simulink model "MicrogridControl"  (R2025b)
settings: Solver=VariableStepAuto  StartTime=0.0  StopTime=8  FixedStep=Ts  RelTol=1e-3
PreLoadFcn:
  | NormalOperation;
  | MicrogridControlParam;
undefined symbols (not defined in the file): base, bessModeInitial, bessSystem, bessVoltage, breakerStatus, DiscIntNeverNeededParam, ee_sli_rtmsupport, event, gcbh, generator, gflInverter, gfmInverter, Inertia, lineInductance, lineResistance, machine, plannedIsland, pmsm, powerLimit, powerQuality, PV, PVInverter, ref, resync, solar, solarInsolationChange, systemFrequency, Ts, windController, windSystem, windTurbine
libraries: nesl_utility x234, ee_lib x174, fl_lib x143, eeGeneralControl x137, simulink x78, eeTransforms x47, slpidlib x23, nesl_utility_internal x12, eePwmGenerator x9, eeSinusoidalMeasurementV2 x9, custom_lib x7, batteryecm_lib x6
(part 24 of 25)

== system MicrogridControl/Solar/Solar Plant Integrated1/Detailed/PV Plant & Controller/Controller/Power Reference/Power Reference Controller/Power Reference Controller/Current_controller ==
  id-ref : Inport
  ipvd : Inport  Port=2
  iqref : Inport  Port=3
  iq : Inport  Port=4
  Vd : Inport  Port=5
  Vq : Inport  Port=6
  Constant4 : Constant  Value=0
  Gain1 : Gain  Gain=2*1*pi*60*L/zbase
  Gain2 : Gain  Gain=2*1*pi*60*L/zbase
  Mux1 : Mux  Inputs=3
  PID Controller : slpidlib/PID Controller  Controller=PID  Form=Parallel  TimeDomain=Discrete-time  UseExternalTs=off  SampleTime=-1  IntegratorMethod=Forward Euler  FilterMethod=Forward Euler  ControllerParametersSource=internal  P=Kpic  I=Kiic  UseKiTs=off  D=Kd  UseExternalDerivativeSource=off  N=100  UseFilter=on  TunerSelectOption=Transfer Function Based (PID Tuner App)  InitialConditionSource=internal  InitialConditionForIntegrator=0  InitialConditionForFilter=0  DifferentiatorICPrevScaledInput=0  ExternalReset=none  TrackingMode=off  Kt=1  LimitOutput=on  SatLimitsSource=internal  UpperSaturationLimit=3  LowerSaturationLimit=-3  LinearizeAsGain=on  AntiWindupMode=clamping  Kb=1  LimitIntegrator=on  UpperIntegratorSaturationLimit=3  LowerIntegratorSaturationLimit=-3  POutMin=[]  POutMax=[]  IOutMin=[]  IOutMax=[]  DOutMin=[]  DOutMax=[]  NOutMin=[]  NOutMax=[]  SumOutMin=[]  SumOutMax=[]  SaturationOutMin=[]  SaturationOutMax=[]  PParamMin=[]  PParamMax=[]  IParamMin=[]  IParamMax=[]  DParamMin=[]  DParamMax=[]  NParamMin=[]  NParamMax=[]  KbParamMin=[]  KbParamMax=[]  KtParamMin=[]  KtParamMax=[]  KbOutMin=[]  KbOutMax=[]  KtOutMin=[]  KtOutMax=[]  IntegratorOutMin=[]  IntegratorOutMax=[]  FilterOutMin=[]  FilterOutMax=[]  SumI1OutMin=[]  SumI1OutMax=[]  SumI2OutMin=[]  SumI2OutMax=[]  SumI3OutMin=[]  SumI3OutMax=[]  SumI4OutMin=[]  SumI4OutMax=[]  SumDOutMin=[]  SumDOutMax=[]  DifferentiatorOutMin=[]  DifferentiatorOutMax=[]  FilterDiffOutCoefMin=[]  FilterDiffOutCoefMax=[]  ReciprocalOutMin=[]  ReciprocalOutMax=[]  SumDenOutMin=[]  SumDenOutMax=[]  SumNumOutMin=[]  SumNumOutMax=[]  DivideOutMin=[]  DivideOutMax=[]  UdiffTsProdOutMin=[]  UdiffTsProdOutMax=[]  NTsProdOutMin=[]  NTsProdOutMax=[]  UintegralTsProdOutMin=[]  UintegralTsProdOutMax=[]  UngainTsProdOutMin=[]  UngainTsProdOutMax=[]  ClampingZeroOutDataTypeStr=Inherit: Inherit via back propagation  ClampingZeroOutMin=[]  ClampingZeroOutMax=[]  FilterDenConstantOutDataTypeStr=Inherit: Inherit via back propagation  FilterDenConstantOutMin=[]  FilterDenConstantOutMax=[]  PCopyOutDataTypeStr=Inherit: Inherit via back propagation  PCopyOutMin=[]  PCopyOutMax=[]  NCopyOutDataTypeStr=Inherit: Inherit via back propagation  NCopyOutMin=[]  NCopyOutMax=[]  IntegratorContinuousStateAttributes=''  IntegratorStateMustResolveToSignalObject=off  IntegratorRTWStateStorageClass=Auto  FilterContinuousStateAttributes=''  FilterStateMustResolveToSignalObject=off  FilterRTWStateStorageClass=Auto  ParallelPVariant=InternalParameters  IdealPVariant=Disabled  IVariant=InternalParameters  DVariant=InternalParameters  IntegratorVariant=Discrete  SatVariant=Enabled  AWVariant=DiscClampingParallel  PCopyVariant=Disabled  TRVariant=Disabled  FdbkBlocksVariant=Forward  IdealPFdbkVariant=Disabled  SatFdbkVariant=Disabled  DerivativeFilterVariant=ForwardEulerFilter  NVariant=InternalParameters  NCopyVariant=Disabled  FilterICVariant=InternalICsFilter  IntegratorICVariant=InternalICs  ExternalResetVariant=Disabled  TRSumVariant=Passthrough  SumFdbkVariant=Disabled  SumVariant=Sum_PID  TsampFilterVariant=InternalTs  TsampNgainVariant=Passthrough  TsampIntegralVariant=Disabled_SignalSpec  ExternalSaturationOutDataTypeStr=Inherit: Same as second input  DerivativeSourceVariant=ErrorSignal  PreIntVariant=InternalPreInt
  PID Controller1 : slpidlib/PID Controller  Controller=PID  Form=Parallel  TimeDomain=Discrete-time  UseExternalTs=off  SampleTime=-1  IntegratorMethod=Forward Euler  FilterMethod=Forward Euler  ControllerParametersSource=internal  P=Kpic  I=Kiic  UseKiTs=off  D=Kd  UseExternalDerivativeSource=off  N=100  UseFilter=on  TunerSelectOption=Transfer Function Based (PID Tuner App)  InitialConditionSource=internal  InitialConditionForIntegrator=0  InitialConditionForFilter=0  DifferentiatorICPrevScaledInput=0  ExternalReset=none  TrackingMode=off  Kt=1  LimitOutput=on  SatLimitsSource=internal  UpperSaturationLimit=3  LowerSaturationLimit=-3  LinearizeAsGain=on  AntiWindupMode=clamping  Kb=1  LimitIntegrator=on  UpperIntegratorSaturationLimit=3  LowerIntegratorSaturationLimit=-3  POutMin=[]  POutMax=[]  IOutMin=[]  IOutMax=[]  DOutMin=[]  DOutMax=[]  NOutMin=[]  NOutMax=[]  SumOutMin=[]  SumOutMax=[]  SaturationOutMin=[]  SaturationOutMax=[]  PParamMin=[]  PParamMax=[]  IParamMin=[]  IParamMax=[]  DParamMin=[]  DParamMax=[]  NParamMin=[]  NParamMax=[]  KbParamMin=[]  KbParamMax=[]  KtParamMin=[]  KtParamMax=[]  KbOutMin=[]  KbOutMax=[]  KtOutMin=[]  KtOutMax=[]  IntegratorOutMin=[]  IntegratorOutMax=[]  FilterOutMin=[]  FilterOutMax=[]  SumI1OutMin=[]  SumI1OutMax=[]  SumI2OutMin=[]  SumI2OutMax=[]  SumI3OutMin=[]  SumI3OutMax=[]  SumI4OutMin=[]  SumI4OutMax=[]  SumDOutMin=[]  SumDOutMax=[]  DifferentiatorOutMin=[]  DifferentiatorOutMax=[]  FilterDiffOutCoefMin=[]  FilterDiffOutCoefMax=[]  ReciprocalOutMin=[]  ReciprocalOutMax=[]  SumDenOutMin=[]  SumDenOutMax=[]  SumNumOutMin=[]  SumNumOutMax=[]  DivideOutMin=[]  DivideOutMax=[]  UdiffTsProdOutMin=[]  UdiffTsProdOutMax=[]  NTsProdOutMin=[]  NTsProdOutMax=[]  UintegralTsProdOutMin=[]  UintegralTsProdOutMax=[]  UngainTsProdOutMin=[]  UngainTsProdOutMax=[]  ClampingZeroOutDataTypeStr=Inherit: Inherit via back propagation  ClampingZeroOutMin=[]  ClampingZeroOutMax=[]  FilterDenConstantOutDataTypeStr=Inherit: Inherit via back propagation  FilterDenConstantOutMin=[]  FilterDenConstantOutMax=[]  PCopyOutDataTypeStr=Inherit: Inherit via back propagation  PCopyOutMin=[]  PCopyOutMax=[]  NCopyOutDataTypeStr=Inherit: Inherit via back propagation  NCopyOutMin=[]  NCopyOutMax=[]  IntegratorContinuousStateAttributes=''  IntegratorStateMustResolveToSignalObject=off  IntegratorRTWStateStorageClass=Auto  FilterContinuousStateAttributes=''  FilterStateMustResolveToSignalObject=off  FilterRTWStateStorageClass=Auto  ParallelPVariant=InternalParameters  IdealPVariant=Disabled  IVariant=InternalParameters  DVariant=InternalParameters  IntegratorVariant=Discrete  SatVariant=Enabled  AWVariant=DiscClampingParallel  PCopyVariant=Disabled  TRVariant=Disabled  FdbkBlocksVariant=Forward  IdealPFdbkVariant=Disabled  SatFdbkVariant=Disabled  DerivativeFilterVariant=ForwardEulerFilter  NVariant=InternalParameters  NCopyVariant=Disabled  FilterICVariant=InternalICsFilter  IntegratorICVariant=InternalICs  ExternalResetVariant=Disabled  TRSumVariant=Passthrough  SumFdbkVariant=Disabled  SumVariant=Sum_PID  TsampFilterVariant=InternalTs  TsampNgainVariant=Passthrough  TsampIntegralVariant=Disabled_SignalSpec  ExternalSaturationOutDataTypeStr=Inherit: Same as second input  DerivativeSourceVariant=ErrorSignal  PreIntVariant=InternalPreInt
  Saturation : Saturate  UpperLimit=1.2  LowerLimit=-1.2
  Saturation1 : Saturate  UpperLimit=1.2  LowerLimit=-1.2
  Scope : Scope  NumInputPorts=2
      settings: ActiveDisplayYMinimum=0.49995  ActiveDisplayYMaximum=0.50039
  Scope1 : Scope  NumInputPorts=2
      settings: ActiveDisplayYMinimum=-1  ActiveDisplayYMaximum=1  DataLoggingVariableName=ScopeData2
  Scope2 : Scope  NumInputPorts=3
      settings: ActiveDisplayYMinimum=0.92426  ActiveDisplayYMaximum=1.0261  DataLoggingVariableName=ScopeData2
  Sum1 : Sum  Inputs=|+-
  Sum3 : Sum  Inputs=|++-
  Sum4 : Sum  Inputs=|+++
  Sum5 : Sum  Inputs=|+-
  mdq0 : Outport
  wires:
  Vd/1 -> Sum3/1, Scope2/1
  Saturation1/1 -> Mux1/2
  Saturation/1 -> Mux1/1
  iqref/1 -> Sum5/1, Scope1/1
  Mux1/1 -> mdq0/1
  Sum4/1 -> [Eq], Saturation1/1
  PID Controller1/1 -> Sum4/1
  Sum5/1 -> PID Controller1/1
  Constant4/1 -> Mux1/3
  Sum1/1 -> PID Controller/1
  iq/1 -> Sum5/2, Gain2/1, Scope1/2
  Vq/1 -> Sum4/2
  Gain1/1 -> Sum4/3
  id-ref/1 -> Sum1/1, Scope/1
  ipvd/1 -> Sum1/2, Gain1/1, Scope/2
  Gain2/1 -> Sum3/3, Scope2/3
  Sum3/1 -> [Ed], Saturation/1
  PID Controller/1 -> Sum3/2, Scope2/2

== system MicrogridControl/Solar/Solar Plant Integrated1/Detailed/PV Plant & Controller/Controller/Power Reference/Power Reference Controller/Power Reference Controller/Reference Current ==
  note: Avoid division by zero during start
  note: Current Limiters
  V-mag : Inport
  LVRT_iq : Inport  Port=2
  PRef : Inport  Port=3
  QRef : Inport  Port=4
  Constant1 : Constant
  Constant3 : Constant  Value=Imax
  Current limits : Subsystem
  Refernce id generation : Subsystem
  Refernce iq generation : Subsystem
  Switch : Switch  Criteria=u2 ~= 0  SaturateOnIntegerOverflow=off  InputSameDT=off
  Unit Delay1 : UnitDelay  SampleTime=Ts  HasFrameUpgradeWarning=on
  Unit Delay3 : UnitDelay  SampleTime=Ts  HasFrameUpgradeWarning=on
  id_ref : Outport
  iq_ref : Outport  Port=2
  wires:
  Current limits/2(iubd) -> Refernce id generation/2(ubid)
  PRef/1 -> Refernce id generation/3(PRef)
  QRef/1 -> Refernce iq generation/4(Q_ref)
  Constant1/1 -> Switch/3
  Switch/1 -> Refernce iq generation/2(V_mag), Refernce id generation/1(V_mag)
  V-mag/1 -> Switch/2, Switch/1
  LVRT_iq/1 -> Refernce iq generation/3(LVRT_iq)
  Refernce iq generation/1(iq_ref) -> iq_ref/1, Unit Delay1/1
  Refernce id generation/1(id_ref) -> Unit Delay3/1, id_ref/1
  Constant3/1 -> Current limits/1(Imax)
  Unit Delay3/1 -> Current limits/3(idref)
  Current limits/1(iubq) -> Refernce iq generation/1(ubiq)
  Unit Delay1/1 -> Current limits/2(iqref)

== system MicrogridControl/Wind Farm/Wind Plant Integrated/Detailed/Wind Turbine and Converters/Wind Controller/Wind Grid-side Converter Controller/DC voltage controller & current reference/Subsystem1/V_dc_Controller1 ==
  Wind_plant1 : Inport
  In2 : Inport  Port=2
  Gain : Gain  Gain=1/Vdc
  PI : Subsystem
  Sum : Sum  Inputs=|+-
  Out1 : Outport
  wires:
  PI/1(Out2) -> Out1/1
  Gain/1 -> PI/1(Input)
  Sum/1 -> Gain/1
  In2/1 -> Sum/2
  Wind_plant1/1 -> Sum/1

== system MicrogridControl/Wind Farm/Wind Plant Integrated/Detailed/Wind Turbine and Converters/Wind Plant/Back-to-Back Converters/Switching/Grid Side Converter/Pulse Generation1 ==
  G : Inport
  Constant : Constant  Value=5
  Subtract : Sum  Inputs=-+
  G1 : Outport  VectorParamsAs1DForOutWhenUnconnected=off
  G2 : Outport  Port=2  VectorParamsAs1DForOutWhenUnconnected=off
  wires:
  G/1 -> Subtract/1, G1/1
  Constant/1 -> Subtract/2
  Subtract/1 -> G2/1

== system MicrogridControl/Wind Farm/Wind Plant Integrated/Detailed/Wind Turbine and Converters/Wind Plant/Back-to-Back Converters/Switching/Machine Side Converter/Pulse Generation ==
  G : Inport
  Constant : Constant  Value=5
  Subtract : Sum  Inputs=-+
  G1 : Outport  VectorParamsAs1DForOutWhenUnconnected=off
  G2 : Outport  Port=2  VectorParamsAs1DForOutWhenUnconnected=off
  wires:
  G/1 -> Subtract/1, G1/1
  Constant/1 -> Subtract/2
  Subtract/1 -> G2/1

== system MicrogridControl/Wind Farm/Wind Plant Integrated1/Detailed/Wind Turbine and Converters/Wind Controller/Wind Grid-side Converter Controller/DC voltage controller & current reference/Subsystem1/V_dc_Controller1 ==
  Wind_plant1 : Inport
  In2 : Inport  Port=2
  Gain : Gain  Gain=1/Vdc
  PI : Subsystem
  Sum : Sum  Inputs=|+-
  Out1 : Outport
  wires:
  PI/1(Out2) -> Out1/1
  Gain/1 -> PI/1(Input)
  Sum/1 -> Gain/1
  In2/1 -> Sum/2
  Wind_plant1/1 -> Sum/1

== system MicrogridControl/Wind Farm/Wind Plant Integrated1/Detailed/Wind Turbine and Converters/Wind Plant/Back-to-Back Converters/Switching/Grid Side Converter/Pulse Generation1 ==
  G : Inport
  Constant : Constant  Value=5
  Subtract : Sum  Inputs=-+
  G1 : Outport  VectorParamsAs1DForOutWhenUnconnected=off
  G2 : Outport  Port=2  VectorParamsAs1DForOutWhenUnconnected=off
  wires:
  G/1 -> Subtract/1, G1/1
  Constant/1 -> Subtract/2
  Subtract/1 -> G2/1

== system MicrogridControl/Wind Farm/Wind Plant Integrated1/Detailed/Wind Turbine and Converters/Wind Plant/Back-to-Back Converters/Switching/Machine Side Converter/Pulse Generation ==
  G : Inport
  Constant : Constant  Value=5
  Subtract : Sum  Inputs=-+
  G1 : Outport  VectorParamsAs1DForOutWhenUnconnected=off
  G2 : Outport  Port=2  VectorParamsAs1DForOutWhenUnconnected=off
  wires:
  G/1 -> Subtract/1, G1/1
  Constant/1 -> Subtract/2
  Subtract/1 -> G2/1

== system MicrogridControl/BESS/BESS Integrated/Detailed/BESS Controller/Grid Forming/Current Limiting/CurrentLimitingMethod/currentLimitAndVirtual/Current Saturation/Compare ==
  u : Inport
  Compare To Zero : simulink/Logic and Bit Operations/Compare To Zero  relop=<=  OutDataTypeStr=boolean
  Data Type Conversion : DataTypeConversion  SaturateOnIntegerOverflow=off  RndMeth=Floor
  Out1 : Outport
  wires:
  Data Type Conversion/1 -> Out1/1
  u/1 -> Compare To Zero/1
  Compare To Zero/1 -> Data Type Conversion/1

== system MicrogridControl/BESS/BESS Integrated/Detailed/BESS Controller/Grid Forming/Current Limiting/CurrentLimitingMethod/currentLimitAndVirtual/Current Saturation/If Action Subsystem ==
  Is : Inport
  Isd : Inport  Port=2
  Isq : Inport  Port=3
  maxI : Inport  Port=4
  Action Port : ActionPort
  Divide : Product  Inputs=*/
  Product : Product
  Product1 : Product
  Idmax : Outport
  Iqmax : Outport  Port=2
  wires:
  Product/1 -> Iqmax/1
  Product1/1 -> Idmax/1
  Isq/1 -> Product/2
  Isd/1 -> Product1/1
  Divide/1 -> Product/1, Product1/2
  Is/1 -> Divide/2
  maxI/1 -> Divide/1

== system MicrogridControl/BESS/BESS Integrated/Detailed/BESS Controller/Grid Forming/Current Limiting/CurrentLimitingMethod/currentLimitAndVirtual/Current Saturation/If Action Subsystem1 ==
  Action Port : ActionPort
  Constant3 : Constant  Value=0
  Constant4 : Constant  Value=0
  Idmax : Outport
  Iqmax : Outport  Port=2
  wires:
  Constant3/1 -> Idmax/1
  Constant4/1 -> Iqmax/1

== system MicrogridControl/BESS/BESS Integrated/Detailed/BESS Controller/Grid Forming/Measurement/Frequency Measurement/Frequency Measurement/If Action Subsystem/Frequency estimation ==
  sk : Inport
  sk-1 : Inport  Port=2
  k : Inport  Port=3
  k-1 : Inport  Port=4
  Trigger : TriggerPort  VariantControl=(inherit)  InitialTriggerSignalState=positive
  Add1 : Sum  Inputs=+-  OutDataTypeStr=double  AccumDataTypeStr=double  RndMeth=Convergent
  Add2 : Sum
  Constant : Constant
  Delay : Delay  DelayLength=1
  Delay1 : Delay  DelayLength=1
  Divide : Product  Inputs=*/  RndMeth=Ceiling
  Gain : Gain  Gain=2  ParamDataTypeStr=double  RndMeth=Convergent
  Gain2 : Gain  Gain=0.5
  MATLAB Function : MATLAB Function  TreatAsAtomicUnit=on
  f : Outport
  wires:
  sk-1/1 -> MATLAB Function/2(y2)
  sk/1 -> MATLAB Function/1(y1)
  k-1/1 -> MATLAB Function/4(x2)  "x1"
  k/1 -> MATLAB Function/3(x1)
  Delay/1 -> Add1/2
  Gain2/1 -> f/1
  Add2/1 -> Gain2/1
  Delay1/1 -> Add2/2
  Divide/1 -> Delay1/1, Add2/1
  MATLAB Function/1(x) -> Add1/1, Delay/1  "x1-y1/slope"
  Gain/1 -> Divide/2
  Constant/1 -> Divide/1
  Add1/1 -> Gain/1

== system MicrogridControl/BESS/BESS Integrated/Detailed/BESS Controller/Grid Forming/Power Control/ActivePowerControl/vsmControl/Damping Frequency/ConstantFreqReference ==
  fref : Inport
  Constant1 : Constant
  Terminator : Terminator
  fmeas : Outport
  wires:
  fref/1 -> Terminator/1
  Constant1/1 -> fmeas/1

== system MicrogridControl/BESS/BESS Integrated/Detailed/BESS Controller/Grid Forming/Power Control/ActivePowerControl/vsmControl/Damping Frequency/WithFrequencyMeasurement ==
  fref : Inport
  fmeas : Outport
  wires:
  fref/1 -> fmeas/1

== system MicrogridControl/BESS/BESS Integrated/Detailed/BESS Controller/Grid Forming/Power Control/ActivePowerControl/vsmControl/Power Reference Selection/If Action Subsystem ==
  note: Frequency difference power
  Pref : Inport
  Wsm : Inport  Port=2
  Action Port : ActionPort  ActionPortLabel=if(u1 > 0)
  Constant : Constant
  Gain6 : Gain  Gain=vsmFreqDroop
  Sum : Sum  Inputs=|+-
  Sum3 : Sum  Inputs=++|
  Power : Outport
  wires:
  Sum3/1 -> Power/1
  Constant/1 -> Sum/1
  Sum/1 -> Gain6/1
  Wsm/1 -> Sum/2
  Pref/1 -> Sum3/1  "Reference power"
  Gain6/1 -> Sum3/2

== system MicrogridControl/BESS/BESS Integrated/Detailed/BESS Controller/Grid Forming/Power Control/ActivePowerControl/vsmControl/Power Reference Selection/If Action Subsystem1 ==
  note: Frequency difference power
  fref : Inport
  Wsm : Inport  Port=2
  Action Port : ActionPort  ActionPortLabel=else
  Gain6 : Gain  Gain=vsmFreqDroop
  Scope : Scope
      settings: ActiveDisplayYMinimum=0.99966  ActiveDisplayYMaximum=1.00057  DataLoggingVariableName=ScopeData14
  Scope1 : Scope
      settings: DataLoggingVariableName=ScopeData15
  Sum : Sum  Inputs=|+-
  Power : Outport
  wires:
  Gain6/1 -> Power/1, Scope1/1
  fref/1 -> Sum/1
  Sum/1 -> Gain6/1
  Wsm/1 -> Sum/2, Scope/1

== system MicrogridControl/BESS/BESS Integrated1/Detailed/BESS Controller/Grid Forming/Current Limiting/CurrentLimitingMethod/currentLimitAndVirtual/Current Saturation/Compare ==
  u : Inport
  Compare To Zero : simulink/Logic and Bit Operations/Compare To Zero  relop=<=  OutDataTypeStr=boolean
  Data Type Conversion : DataTypeConversion  SaturateOnIntegerOverflow=off  RndMeth=Floor
  Out1 : Outport
  wires:
  Data Type Conversion/1 -> Out1/1
  u/1 -> Compare To Zero/1
  Compare To Zero/1 -> Data Type Conversion/1

== system MicrogridControl/BESS/BESS Integrated1/Detailed/BESS Controller/Grid Forming/Current Limiting/CurrentLimitingMethod/currentLimitAndVirtual/Current Saturation/If Action Subsystem ==
  Is : Inport
  Isd : Inport  Port=2
  Isq : Inport  Port=3
  maxI : Inport  Port=4
  Action Port : ActionPort
  Divide : Product  Inputs=*/
  Product : Product
  Product1 : Product
  Idmax : Outport
  Iqmax : Outport  Port=2
  wires:
  Product/1 -> Iqmax/1
  Product1/1 -> Idmax/1
  Isq/1 -> Product/2
  Isd/1 -> Product1/1
  Divide/1 -> Product/1, Product1/2
  Is/1 -> Divide/2
  maxI/1 -> Divide/1

== system MicrogridControl/BESS/BESS Integrated1/Detailed/BESS Controller/Grid Forming/Current Limiting/CurrentLimitingMethod/currentLimitAndVirtual/Current Saturation/If Action Subsystem1 ==
  Action Port : ActionPort
  Constant3 : Constant  Value=0
  Constant4 : Constant  Value=0
  Idmax : Outport
  Iqmax : Outport  Port=2
  wires:
  Constant3/1 -> Idmax/1
  Constant4/1 -> Iqmax/1

== system MicrogridControl/BESS/BESS Integrated1/Detailed/BESS Controller/Grid Forming/Measurement/Frequency Measurement/Frequency Measurement/If Action Subsystem/Frequency estimation ==
  sk : Inport
  sk-1 : Inport  Port=2
  k : Inport  Port=3
  k-1 : Inport  Port=4
  Trigger : TriggerPort  VariantControl=(inherit)  InitialTriggerSignalState=positive
  Add1 : Sum  Inputs=+-  OutDataTypeStr=double  AccumDataTypeStr=double  RndMeth=Convergent
  Add2 : Sum
  Constant : Constant
  Delay : Delay  DelayLength=1
  Delay1 : Delay  DelayLength=1
  Divide : Product  Inputs=*/  RndMeth=Ceiling
  Gain : Gain  Gain=2  ParamDataTypeStr=double  RndMeth=Convergent
  Gain2 : Gain  Gain=0.5
  MATLAB Function : MATLAB Function  TreatAsAtomicUnit=on
  f : Outport
  wires:
  sk-1/1 -> MATLAB Function/2(y2)
  sk/1 -> MATLAB Function/1(y1)
  k-1/1 -> MATLAB Function/4(x2)  "x1"
  k/1 -> MATLAB Function/3(x1)
  Delay/1 -> Add1/2
  Gain2/1 -> f/1
  Add2/1 -> Gain2/1
  Delay1/1 -> Add2/2
  Divide/1 -> Delay1/1, Add2/1
  MATLAB Function/1(x) -> Add1/1, Delay/1  "x1-y1/slope"
  Gain/1 -> Divide/2
  Constant/1 -> Divide/1
  Add1/1 -> Gain/1

== system MicrogridControl/BESS/BESS Integrated1/Detailed/BESS Controller/Grid Forming/Power Control/ActivePowerControl/vsmControl/Damping Frequency/ConstantFreqReference ==
  fref : Inport
  Constant1 : Constant
  Terminator : Terminator
  fmeas : Outport
  wires:
  fref/1 -> Terminator/1
  Constant1/1 -> fmeas/1

== system MicrogridControl/BESS/BESS Integrated1/Detailed/BESS Controller/Grid Forming/Power Control/ActivePowerControl/vsmControl/Damping Frequency/WithFrequencyMeasurement ==
  fref : Inport
  fmeas : Outport
  wires:
  fref/1 -> fmeas/1

== system MicrogridControl/BESS/BESS Integrated1/Detailed/BESS Controller/Grid Forming/Power Control/ActivePowerControl/vsmControl/Power Reference Selection/If Action Subsystem ==
  note: Frequency difference power
  Pref : Inport
  Wsm : Inport  Port=2
  Action Port : ActionPort  ActionPortLabel=if(u1 > 0)
  Constant : Constant
  Gain6 : Gain  Gain=vsmFreqDroop
  Sum : Sum  Inputs=|+-
  Sum3 : Sum  Inputs=++|
  Power : Outport
  wires:
  Sum3/1 -> Power/1
  Constant/1 -> Sum/1
  Sum/1 -> Gain6/1
  Wsm/1 -> Sum/2
  Pref/1 -> Sum3/1  "Reference power"
  Gain6/1 -> Sum3/2

== system MicrogridControl/BESS/BESS Integrated1/Detailed/BESS Controller/Grid Forming/Power Control/ActivePowerControl/vsmControl/Power Reference Selection/If Action Subsystem1 ==
  note: Frequency difference power
  fref : Inport
  Wsm : Inport  Port=2
  Action Port : ActionPort  ActionPortLabel=else
  Gain6 : Gain  Gain=vsmFreqDroop
  Scope : Scope
      settings: ActiveDisplayYMinimum=0.99966  ActiveDisplayYMaximum=1.00057  DataLoggingVariableName=ScopeData14
  Scope1 : Scope
      settings: DataLoggingVariableName=ScopeData15
  Sum : Sum  Inputs=|+-
  Power : Outport
  wires:
  Gain6/1 -> Power/1, Scope1/1
  fref/1 -> Sum/1
  Sum/1 -> Gain6/1
  Wsm/1 -> Sum/2, Scope/1

== system MicrogridControl/BESS/BESS Integrated3/Detailed/BESS Controller/Grid Forming/Current Limiting/CurrentLimitingMethod/currentLimitAndVirtual/Current Saturation/Compare ==
  u : Inport
  Compare To Zero : simulink/Logic and Bit Operations/Compare To Zero  relop=<=  OutDataTypeStr=boolean
  Data Type Conversion : DataTypeConversion  SaturateOnIntegerOverflow=off  RndMeth=Floor
  Out1 : Outport
  wires:
  Data Type Conversion/1 -> Out1/1
  u/1 -> Compare To Zero/1
  Compare To Zero/1 -> Data Type Conversion/1

== system MicrogridControl/BESS/BESS Integrated3/Detailed/BESS Controller/Grid Forming/Current Limiting/CurrentLimitingMethod/currentLimitAndVirtual/Current Saturation/If Action Subsystem ==
  Is : Inport
  Isd : Inport  Port=2
  Isq : Inport  Port=3
  maxI : Inport  Port=4
  Action Port : ActionPort
  Divide : Product  Inputs=*/
  Product : Product
  Product1 : Product
  Idmax : Outport
  Iqmax : Outport  Port=2
  wires:
  Product/1 -> Iqmax/1
  Product1/1 -> Idmax/1
  Isq/1 -> Product/2
  Isd/1 -> Product1/1
  Divide/1 -> Product/1, Product1/2
  Is/1 -> Divide/2
  maxI/1 -> Divide/1

== system MicrogridControl/BESS/BESS Integrated3/Detailed/BESS Controller/Grid Forming/Current Limiting/CurrentLimitingMethod/currentLimitAndVirtual/Current Saturation/If Action Subsystem1 ==
  Action Port : ActionPort
  Constant3 : Constant  Value=0
  Constant4 : Constant  Value=0
  Idmax : Outport
  Iqmax : Outport  Port=2
  wires:
  Constant3/1 -> Idmax/1
  Constant4/1 -> Iqmax/1

== system MicrogridControl/BESS/BESS Integrated3/Detailed/BESS Controller/Grid Forming/Measurement/Frequency Measurement/Frequency Measurement/If Action Subsystem/Frequency estimation ==
  sk : Inport
  sk-1 : Inport  Port=2
  k : Inport  Port=3
  k-1 : Inport  Port=4
  Trigger : TriggerPort  VariantControl=(inherit)  InitialTriggerSignalState=positive
  Add1 : Sum  Inputs=+-  OutDataTypeStr=double  AccumDataTypeStr=double  RndMeth=Convergent
  Add2 : Sum
  Constant : Constant
  Delay : Delay  DelayLength=1
  Delay1 : Delay  DelayLength=1
  Divide : Product  Inputs=*/  RndMeth=Ceiling
  Gain : Gain  Gain=2  ParamDataTypeStr=double  RndMeth=Convergent
  Gain2 : Gain  Gain=0.5
  MATLAB Function : MATLAB Function  TreatAsAtomicUnit=on
  f : Outport
  wires:
  sk-1/1 -> MATLAB Function/2(y2)
  sk/1 -> MATLAB Function/1(y1)
  k-1/1 -> MATLAB Function/4(x2)  "x1"
  k/1 -> MATLAB Function/3(x1)
  Delay/1 -> Add1/2
  Gain2/1 -> f/1
  Add2/1 -> Gain2/1
  Delay1/1 -> Add2/2
  Divide/1 -> Delay1/1, Add2/1
  MATLAB Function/1(x) -> Add1/1, Delay/1  "x1-y1/slope"
  Gain/1 -> Divide/2
  Constant/1 -> Divide/1
  Add1/1 -> Gain/1

== system MicrogridControl/BESS/BESS Integrated3/Detailed/BESS Controller/Grid Forming/Power Control/ActivePowerControl/vsmControl/Damping Frequency/ConstantFreqReference ==
  fref : Inport
  Constant1 : Constant
  Terminator : Terminator
  fmeas : Outport
  wires:
  fref/1 -> Terminator/1
  Constant1/1 -> fmeas/1

== system MicrogridControl/BESS/BESS Integrated3/Detailed/BESS Controller/Grid Forming/Power Control/ActivePowerControl/vsmControl/Damping Frequency/WithFrequencyMeasurement ==
  fref : Inport
  fmeas : Outport
  wires:
  fref/1 -> fmeas/1

== system MicrogridControl/BESS/BESS Integrated3/Detailed/BESS Controller/Grid Forming/Power Control/ActivePowerControl/vsmControl/Power Reference Selection/If Action Subsystem ==
  note: Frequency difference power
  Pref : Inport
  Wsm : Inport  Port=2
  Action Port : ActionPort  ActionPortLabel=if(u1 > 0)
  Constant : Constant
  Gain6 : Gain  Gain=vsmFreqDroop
  Sum : Sum  Inputs=|+-
  Sum3 : Sum  Inputs=++|
  Power : Outport
  wires:
  Sum3/1 -> Power/1
  Constant/1 -> Sum/1
  Sum/1 -> Gain6/1
  Wsm/1 -> Sum/2
  Pref/1 -> Sum3/1  "Reference power"
  Gain6/1 -> Sum3/2

== system MicrogridControl/BESS/BESS Integrated3/Detailed/BESS Controller/Grid Forming/Power Control/ActivePowerControl/vsmControl/Power Reference Selection/If Action Subsystem1 ==
  note: Frequency difference power
  fref : Inport
  Wsm : Inport  Port=2
  Action Port : ActionPort  ActionPortLabel=else
  Gain6 : Gain  Gain=0.5%0.5vsmFreqDroop
  Scope : Scope
      settings: ActiveDisplayYMinimum=-0.12553668206522495  ActiveDisplayYMaximum=1.1298301385870249  DataLoggingVariableName=ScopeData14
  Scope1 : Scope
      settings: ActiveDisplayYMinimum=-1  ActiveDisplayYMaximum=1  DataLoggingVariableName=ScopeData15
  Sum : Sum  Inputs=|+-
  Power : Outport
  wires:
  Gain6/1 -> Power/1, Scope1/1
  fref/1 -> Sum/1
  Sum/1 -> Gain6/1
  Wsm/1 -> Sum/2, Scope/1

== system MicrogridControl/Solar/Solar Plant Integrated/Detailed/PV Plant & Controller/Controller/MPPT/Solar PV Controller/DC voltage controller & current reference/If Action Subsystem/Subsystem ==
  V mag : Inport
  iq ub : Inport  Port=2
  Q ref : Inport  Port=3
  Constant : Constant  Value=1e-3
  Data Type Conversion Inherited : simulink/Signal Attributes/Data Type Conversion Inherited  ConvertRealWorld=Real World Value  DoSatur=off
  Divide2 : Product  Inputs=*/
  Gain3 : Gain  Gain=-1
  Saturation Dynamic2 : simulink/Discontinuities/Saturation Dynamic  OutMin=[]  OutMax=[]  OutDataTypeStr=Inherit: Same as second input  OutDataType=fixdt(1, 16)  OutScaling=2^-10  DoSatur=off
  Switch : Switch  Criteria=u2 ~= 0  SaturateOnIntegerOverflow=off  InputSameDT=off
  iq ub1 : InportShadow  Port=2
  iqref : Outport
  wires:
  Data Type Conversion Inherited/1 -> Switch/3
  Constant/1 -> Data Type Conversion Inherited/2
  Switch/1 -> Divide2/2
  V mag/1 -> Switch/1, Switch/2, Data Type Conversion Inherited/1
  Saturation Dynamic2/1 -> iqref/1
  iq ub/1 -> Saturation Dynamic2/1
  Gain3/1 -> Saturation Dynamic2/3
  Q ref/1 -> Divide2/1
  Divide2/1 -> Saturation Dynamic2/2
  iq ub1/1 -> Gain3/1

== system MicrogridControl/Solar/Solar Plant Integrated/Detailed/PV Plant & Controller/Controller/MPPT/Solar PV Controller/DC voltage controller & current reference/If Action Subsystem/Subsystem1 ==
  Vmag : Inport
  P pv : Inport  Port=2
  vdc : Inport  Port=3
  vdc ref : Inport  Port=4
  id ub : Inport  Port=5
  Constant : Constant  Value=1e-3
  Constant4 : Constant  Value=0
  Data Type Conversion Inherited : simulink/Signal Attributes/Data Type Conversion Inherited  ConvertRealWorld=Real World Value  DoSatur=off
  Divide : Product  Inputs=/*
  Gain4 : Gain  Gain=1/(mVAbase)
  Saturation Dynamic1 : simulink/Discontinuities/Saturation Dynamic  OutMin=[]  OutMax=[]  OutDataTypeStr=Inherit: Same as second input  OutDataType=fixdt(1, 16)  OutScaling=2^-10  DoSatur=off
  Scope : Scope  NumInputPorts=2
      settings: ActiveDisplayYMinimum=-55957.97767  ActiveDisplayYMaximum=503630.2665
  Sum : Sum  Inputs=|++
  Switch : Switch  Criteria=u2 ~= 0  SaturateOnIntegerOverflow=off  InputSameDT=off
  V_dc_Controller1 : Subsystem
  idref : Outport
  wires:
  Data Type Conversion Inherited/1 -> Switch/3
  Constant/1 -> Data Type Conversion Inherited/2
  Switch/1 -> Divide/1
  Vmag/1 -> Switch/1, Switch/2, Data Type Conversion Inherited/1
  vdc/1 -> Scope/1, V_dc_Controller1/1(vdc)
  Saturation Dynamic1/1 -> idref/1
  Divide/1 -> Sum/1
  Gain4/1 -> Divide/2
  id ub/1 -> Saturation Dynamic1/1
  vdc ref/1 -> Scope/2, V_dc_Controller1/2(vdc ref)
  Sum/1 -> Saturation Dynamic1/2
  V_dc_Controller1/1(Out1) -> Sum/2
  P pv/1 -> Gain4/1
  Constant4/1 -> Saturation Dynamic1/3

== system MicrogridControl/Solar/Solar Plant Integrated/Detailed/PV Plant & Controller/Controller/MPPT/Solar PV Controller/DC voltage controller & current reference/Subsystem1/V_dc_Controller1 ==
  vdc : Inport
  vdc ref : Inport  Port=2
  Gain : Gain  Gain=1/VdcBase
  PID Controller : slpidlib/PID Controller  Controller=PID  Form=Parallel  TimeDomain=Discrete-time  UseExternalTs=off  SampleTime=-1  IntegratorMethod=Forward Euler  FilterMethod=Forward Euler  ControllerParametersSource=internal  P=Kpv  I=Kiv  UseKiTs=off  D=Kdv  UseExternalDerivativeSource=off  N=100  UseFilter=on  TunerSelectOption=Transfer Function Based (PID Tuner App)  ZeroCross=off  InitialConditionSource=internal  InitialConditionForIntegrator=0  InitialConditionForFilter=0  DifferentiatorICPrevScaledInput=0  ExternalReset=none  TrackingMode=off  Kt=1  LimitOutput=off  SatLimitsSource=internal  UpperSaturationLimit=iMax  LowerSaturationLimit=0  LinearizeAsGain=on  AntiWindupMode=clamping  Kb=1  LimitIntegrator=off  UpperIntegratorSaturationLimit=inf  LowerIntegratorSaturationLimit=-inf  POutMin=[]  POutMax=[]  IOutMin=[]  IOutMax=[]  DOutMin=[]  DOutMax=[]  NOutMin=[]  NOutMax=[]  SumOutMin=[]  SumOutMax=[]  SaturationOutMin=[]  SaturationOutMax=[]  PParamMin=[]  PParamMax=[]  IParamMin=[]  IParamMax=[]  DParamMin=[]  DParamMax=[]  NParamMin=[]  NParamMax=[]  KbParamMin=[]  KbParamMax=[]  KtParamMin=[]  KtParamMax=[]  KbOutMin=[]  KbOutMax=[]  KtOutMin=[]  KtOutMax=[]  IntegratorOutMin=[]  IntegratorOutMax=[]  FilterOutMin=[]  FilterOutMax=[]  SumI1OutMin=[]  SumI1OutMax=[]  SumI2OutMin=[]  SumI2OutMax=[]  SumI3OutMin=[]  SumI3OutMax=[]  SumI4OutMin=[]  SumI4OutMax=[]  SumDOutMin=[]  SumDOutMax=[]  DifferentiatorOutMin=[]  DifferentiatorOutMax=[]  FilterDiffOutCoefMin=[]  FilterDiffOutCoefMax=[]  ReciprocalOutMin=[]  ReciprocalOutMax=[]  SumDenOutMin=[]  SumDenOutMax=[]  SumNumOutMin=[]  SumNumOutMax=[]  DivideOutMin=[]  DivideOutMax=[]  UdiffTsProdOutMin=[]  UdiffTsProdOutMax=[]  NTsProdOutMin=[]  NTsProdOutMax=[]  UintegralTsProdOutMin=[]  UintegralTsProdOutMax=[]  UngainTsProdOutMin=[]  UngainTsProdOutMax=[]  ClampingZeroOutDataTypeStr=Inherit: Inherit via back propagation  ClampingZeroOutMin=[]  ClampingZeroOutMax=[]  FilterDenConstantOutDataTypeStr=Inherit: Inherit via back propagation  FilterDenConstantOutMin=[]  FilterDenConstantOutMax=[]  PCopyOutDataTypeStr=Inherit: Inherit via back propagation  PCopyOutMin=[]  PCopyOutMax=[]  NCopyOutDataTypeStr=Inherit: Inherit via back propagation  NCopyOutMin=[]  NCopyOutMax=[]  IntegratorContinuousStateAttributes=''  IntegratorStateMustResolveToSignalObject=off  IntegratorRTWStateStorageClass=Auto  FilterContinuousStateAttributes=''  FilterStateMustResolveToSignalObject=off  FilterRTWStateStorageClass=Auto  ParallelPVariant=InternalParameters  IdealPVariant=Disabled  IVariant=InternalParameters  DVariant=InternalParameters  IntegratorVariant=Discrete  SatVariant=Disabled  AWVariant=Passthrough  PCopyVariant=Disabled  TRVariant=Disabled  FdbkBlocksVariant=Forward  IdealPFdbkVariant=Disabled  SatFdbkVariant=Disabled  DerivativeFilterVariant=ForwardEulerFilter  NVariant=InternalParameters  NCopyVariant=Disabled  FilterICVariant=InternalICsFilter  IntegratorICVariant=InternalICs  ExternalResetVariant=Disabled  TRSumVariant=Passthrough  SumFdbkVariant=Disabled  SumVariant=Sum_PID  TsampFilterVariant=InternalTs  TsampNgainVariant=Passthrough  TsampIntegralVariant=Disabled_SignalSpec  ExternalSaturationOutDataTypeStr=Inherit: Same as second input  DerivativeSourceVariant=ErrorSignal  PreIntVariant=InternalPreInt
  Sum : Sum  Inputs=|+-
  Out1 : Outport
  wires:
  Sum/1 -> Gain/1
  Gain/1 -> PID Controller/1
  PID Controller/1 -> Out1/1
  vdc ref/1 -> Sum/2
  vdc/1 -> Sum/1

== system MicrogridControl/Solar/Solar Plant Integrated/Detailed/PV Plant & Controller/Controller/Power Reference/Power Reference Controller/Power Reference Controller/Reference Current/Current limits ==
  Imax : Inport
  iqref : Inport  Port=2
  idref : Inport  Port=3
  Constant8 : Constant  Value=0
  Constant9 : Constant  Value=0
  Scope : Scope
      settings: ActiveDisplayYMinimum=-0.15  ActiveDisplayYMaximum=1.35  DataLoggingVariableName=ScopeData3
  Scope1 : Scope
      settings: ActiveDisplayYMinimum=-0.08298  ActiveDisplayYMaximum=0.74678  DataLoggingVariableName=ScopeData4
  Sqrt : Sqrt
  Sqrt1 : Sqrt
  Square{1..4} (4 alike) : Math  Operator=square
  Step2 : Step  Time=0.01  SampleTime=Ts
  Step3 : Step  Time=0.01  SampleTime=Ts
  Sum6 : Sum  Inputs=|+-
  Sum9 : Sum  Inputs=|+-
  Switch1 : Switch  Threshold=.01  SaturateOnIntegerOverflow=off  InputSameDT=off
  Switch2 : Switch  Threshold=.01  SaturateOnIntegerOverflow=off  InputSameDT=off
  iubq : Outport
  iubd : Outport  Port=2
  wires:
  idref/1 -> Square4/1
  Sqrt1/1 -> iubq/1, Scope1/1
  Imax/1 -> Square1/1, Square3/1
  Sqrt/1 -> iubd/1, Scope/1
  Constant9/1 -> Switch2/3
  Square4/1 -> Sum9/2
  Constant8/1 -> Switch1/3
  Square2/1 -> Sum6/2
  Sum6/1 -> Switch1/1
  Square3/1 -> Sum9/1
  iqref/1 -> Square2/1
  Switch1/1 -> Sqrt/1
  Square1/1 -> Sum6/1
  Switch2/1 -> Sqrt1/1
  Step2/1 -> Switch1/2
  Step3/1 -> Switch2/2
  Sum9/1 -> Switch2/1

== system MicrogridControl/Solar/Solar Plant Integrated/Detailed/PV Plant & Controller/Controller/Power Reference/Power Reference Controller/Power Reference Controller/Reference Current/Refernce id generation ==
  V_mag : Inport
  ubid : Inport  Port=2
  PRef : Inport  Port=3
  Divide : Product  Inputs=/*
  Gain6 : Gain  Gain=-1
  P/Q Priority : Switch  Criteria=u2 ~= 0  SaturateOnIntegerOverflow=off  InputSameDT=off
  Priority Mode : Constant  Value=P-2
  Saturation Dynamic2 : simulink/Discontinuities/Saturation Dynamic  OutMin=[]  OutMax=[]  OutDataTypeStr=Inherit: Same as second input  OutDataType=fixdt(1, 16)  OutScaling=2^-10  DoSatur=off
  Saturation1 : Saturate  UpperLimit=Imax  LowerLimit=-Imax
  Scope : Scope
      settings: ActiveDisplayYMinimum=0.99583  ActiveDisplayYMaximum=1.02853
  Scope1 : Scope
      settings: ActiveDisplayYMinimum=-0.12499  ActiveDisplayYMaximum=1.12489  DataLoggingVariableName=ScopeData2
  ubid1 : InportShadow  Port=2
  id_ref : Outport
  wires:
  Divide/1 -> Saturation1/1, Saturation Dynamic2/2
  V_mag/1 -> Divide/1
  P/Q Priority/1 -> id_ref/1, Scope/1
  ubid1/1 -> Gain6/1
  Saturation1/1 -> P/Q Priority/1
  Priority Mode/1 -> P/Q Priority/2
  Saturation Dynamic2/1 -> P/Q Priority/3, Scope1/1
  Gain6/1 -> Saturation Dynamic2/3
  ubid/1 -> Saturation Dynamic2/1
  PRef/1 -> Divide/2

== system MicrogridControl/Solar/Solar Plant Integrated/Detailed/PV Plant & Controller/Controller/Power Reference/Power Reference Controller/Power Reference Controller/Reference Current/Refernce iq generation ==
  ubiq : Inport
  V_mag : Inport  Port=2
  LVRT_iq : Inport  Port=3
  Q_ref : Inport  Port=4
  Divide1 : Product  Inputs=*/
  Gain : Gain  Gain=-1
  Gain1 : Gain  Gain=-1
  Gain7 : Gain  Gain=-1
  LVRT Priority : Switch  Threshold=.9  SaturateOnIntegerOverflow=off  InputSameDT=off
  P/Q Priority : Switch  Criteria=u2 ~= 0  SaturateOnIntegerOverflow=off  InputSameDT=off
  Priority Mode : Constant  Value=P-2
  Saturation Dynamic : simulink/Discontinuities/Saturation Dynamic  OutMin=[]  OutMax=[]  OutDataTypeStr=Inherit: Same as second input  OutDataType=fixdt(1, 16)  OutScaling=2^-10  DoSatur=off
  Saturation2 : Saturate  UpperLimit=1  LowerLimit=-1
  Saturation3 : Saturate  UpperLimit=Imax  LowerLimit=-Imax
  Scope : Scope  NumInputPorts=3
      settings: ActiveDisplayYMinimum=-0.025  ActiveDisplayYMaximum=0.22499  DataLoggingVariableName=ScopeData10
  ubiq1 : InportShadow
  iq_ref : Outport
  wires:
  Gain/1 -> iq_ref/1
  V_mag/1 -> Divide1/2, LVRT Priority/2
  Q_ref/1 -> Divide1/1
  ubiq1/1 -> Gain7/1
  LVRT_iq/1 -> Saturation2/1
  Gain7/1 -> Saturation Dynamic/3
  Saturation Dynamic/1 -> P/Q Priority/1
  Divide1/1 -> Saturation Dynamic/2, Saturation3/1
  Priority Mode/1 -> P/Q Priority/2
  Saturation3/1 -> P/Q Priority/3
  Saturation2/1 -> Gain1/1
  ubiq/1 -> Saturation Dynamic/1
  Gain1/1 -> LVRT Priority/3
  P/Q Priority/1 -> Scope/1, LVRT Priority/1
  LVRT Priority/1 -> Gain/1

== system MicrogridControl/Solar/Solar Plant Integrated1/Detailed/PV Plant & Controller/Controller/MPPT/Solar PV Controller/DC voltage controller & current reference/If Action Subsystem/Subsystem ==
  V mag : Inport
  iq ub : Inport  Port=2
  Q ref : Inport  Port=3
  Constant : Constant  Value=1e-3
  Data Type Conversion Inherited : simulink/Signal Attributes/Data Type Conversion Inherited  ConvertRealWorld=Real World Value  DoSatur=off
  Divide2 : Product  Inputs=*/
  Gain3 : Gain  Gain=-1
  Saturation Dynamic2 : simulink/Discontinuities/Saturation Dynamic  OutMin=[]  OutMax=[]  OutDataTypeStr=Inherit: Same as second input  OutDataType=fixdt(1, 16)  OutScaling=2^-10  DoSatur=off
  Switch : Switch  Criteria=u2 ~= 0  SaturateOnIntegerOverflow=off  InputSameDT=off
  iq ub1 : InportShadow  Port=2
  iqref : Outport
  wires:
  Data Type Conversion Inherited/1 -> Switch/3
  Constant/1 -> Data Type Conversion Inherited/2
  Switch/1 -> Divide2/2
  V mag/1 -> Switch/1, Switch/2, Data Type Conversion Inherited/1
  Saturation Dynamic2/1 -> iqref/1
  iq ub/1 -> Saturation Dynamic2/1
  Gain3/1 -> Saturation Dynamic2/3
  Q ref/1 -> Divide2/1
  Divide2/1 -> Saturation Dynamic2/2
  iq ub1/1 -> Gain3/1

== system MicrogridControl/Solar/Solar Plant Integrated1/Detailed/PV Plant & Controller/Controller/MPPT/Solar PV Controller/DC voltage controller & current reference/If Action Subsystem/Subsystem1 ==
  Vmag : Inport
  P pv : Inport  Port=2
  vdc : Inport  Port=3
  vdc ref : Inport  Port=4
  id ub : Inport  Port=5
  Constant : Constant  Value=1e-3
  Constant4 : Constant  Value=0
  Data Type Conversion Inherited : simulink/Signal Attributes/Data Type Conversion Inherited  ConvertRealWorld=Real World Value  DoSatur=off
  Divide : Product  Inputs=/*
  Gain4 : Gain  Gain=1/(mVAbase)
  Saturation Dynamic1 : simulink/Discontinuities/Saturation Dynamic  OutMin=[]  OutMax=[]  OutDataTypeStr=Inherit: Same as second input  OutDataType=fixdt(1, 16)  OutScaling=2^-10  DoSatur=off
  Scope : Scope  NumInputPorts=2
      settings: ActiveDisplayYMinimum=-55957.97767  ActiveDisplayYMaximum=503630.2665
  Sum : Sum  Inputs=|++
  Switch : Switch  Criteria=u2 ~= 0  SaturateOnIntegerOverflow=off  InputSameDT=off
  V_dc_Controller1 : Subsystem
  idref : Outport
  wires:
  Data Type Conversion Inherited/1 -> Switch/3
  Constant/1 -> Data Type Conversion Inherited/2
  Switch/1 -> Divide/1
  Vmag/1 -> Switch/1, Switch/2, Data Type Conversion Inherited/1
  vdc/1 -> Scope/1, V_dc_Controller1/1(vdc)
  Saturation Dynamic1/1 -> idref/1
  Divide/1 -> Sum/1
  Gain4/1 -> Divide/2
  id ub/1 -> Saturation Dynamic1/1
  vdc ref/1 -> Scope/2, V_dc_Controller1/2(vdc ref)
  Sum/1 -> Saturation Dynamic1/2
  V_dc_Controller1/1(Out1) -> Sum/2
  P pv/1 -> Gain4/1
  Constant4/1 -> Saturation Dynamic1/3

== system MicrogridControl/Solar/Solar Plant Integrated1/Detailed/PV Plant & Controller/Controller/MPPT/Solar PV Controller/DC voltage controller & current reference/Subsystem1/V_dc_Controller1 ==
  vdc : Inport
  vdc ref : Inport  Port=2
  Gain : Gain  Gain=1/VdcBase
  PID Controller : slpidlib/PID Controller  Controller=PID  Form=Parallel  TimeDomain=Discrete-time  UseExternalTs=off  SampleTime=-1  IntegratorMethod=Forward Euler  FilterMethod=Forward Euler  ControllerParametersSource=internal  P=Kpv  I=Kiv  UseKiTs=off  D=Kdv  UseExternalDerivativeSource=off  N=100  UseFilter=on  TunerSelectOption=Transfer Function Based (PID Tuner App)  ZeroCross=off  InitialConditionSource=internal  InitialConditionForIntegrator=0  InitialConditionForFilter=0  DifferentiatorICPrevScaledInput=0  ExternalReset=none  TrackingMode=off  Kt=1  LimitOutput=off  SatLimitsSource=internal  UpperSaturationLimit=iMax  LowerSaturationLimit=0  LinearizeAsGain=on  AntiWindupMode=clamping  Kb=1  LimitIntegrator=off  UpperIntegratorSaturationLimit=inf  LowerIntegratorSaturationLimit=-inf  POutMin=[]  POutMax=[]  IOutMin=[]  IOutMax=[]  DOutMin=[]  DOutMax=[]  NOutMin=[]  NOutMax=[]  SumOutMin=[]  SumOutMax=[]  SaturationOutMin=[]  SaturationOutMax=[]  PParamMin=[]  PParamMax=[]  IParamMin=[]  IParamMax=[]  DParamMin=[]  DParamMax=[]  NParamMin=[]  NParamMax=[]  KbParamMin=[]  KbParamMax=[]  KtParamMin=[]  KtParamMax=[]  KbOutMin=[]  KbOutMax=[]  KtOutMin=[]  KtOutMax=[]  IntegratorOutMin=[]  IntegratorOutMax=[]  FilterOutMin=[]  FilterOutMax=[]  SumI1OutMin=[]  SumI1OutMax=[]  SumI2OutMin=[]  SumI2OutMax=[]  SumI3OutMin=[]  SumI3OutMax=[]  SumI4OutMin=[]  SumI4OutMax=[]  SumDOutMin=[]  SumDOutMax=[]  DifferentiatorOutMin=[]  DifferentiatorOutMax=[]  FilterDiffOutCoefMin=[]  FilterDiffOutCoefMax=[]  ReciprocalOutMin=[]  ReciprocalOutMax=[]  SumDenOutMin=[]  SumDenOutMax=[]  SumNumOutMin=[]  SumNumOutMax=[]  DivideOutMin=[]  DivideOutMax=[]  UdiffTsProdOutMin=[]  UdiffTsProdOutMax=[]  NTsProdOutMin=[]  NTsProdOutMax=[]  UintegralTsProdOutMin=[]  UintegralTsProdOutMax=[]  UngainTsProdOutMin=[]  UngainTsProdOutMax=[]  ClampingZeroOutDataTypeStr=Inherit: Inherit via back propagation  ClampingZeroOutMin=[]  ClampingZeroOutMax=[]  FilterDenConstantOutDataTypeStr=Inherit: Inherit via back propagation  FilterDenConstantOutMin=[]  FilterDenConstantOutMax=[]  PCopyOutDataTypeStr=Inherit: Inherit via back propagation  PCopyOutMin=[]  PCopyOutMax=[]  NCopyOutDataTypeStr=Inherit: Inherit via back propagation  NCopyOutMin=[]  NCopyOutMax=[]  IntegratorContinuousStateAttributes=''  IntegratorStateMustResolveToSignalObject=off  IntegratorRTWStateStorageClass=Auto  FilterContinuousStateAttributes=''  FilterStateMustResolveToSignalObject=off  FilterRTWStateStorageClass=Auto  ParallelPVariant=InternalParameters  IdealPVariant=Disabled  IVariant=InternalParameters  DVariant=InternalParameters  IntegratorVariant=Discrete  SatVariant=Disabled  AWVariant=Passthrough  PCopyVariant=Disabled  TRVariant=Disabled  FdbkBlocksVariant=Forward  IdealPFdbkVariant=Disabled  SatFdbkVariant=Disabled  DerivativeFilterVariant=ForwardEulerFilter  NVariant=InternalParameters  NCopyVariant=Disabled  FilterICVariant=InternalICsFilter  IntegratorICVariant=InternalICs  ExternalResetVariant=Disabled  TRSumVariant=Passthrough  SumFdbkVariant=Disabled  SumVariant=Sum_PID  TsampFilterVariant=InternalTs  TsampNgainVariant=Passthrough  TsampIntegralVariant=Disabled_SignalSpec  ExternalSaturationOutDataTypeStr=Inherit: Same as second input  DerivativeSourceVariant=ErrorSignal  PreIntVariant=InternalPreInt
  Sum : Sum  Inputs=|+-
  Out1 : Outport
  wires:
  Sum/1 -> Gain/1
  Gain/1 -> PID Controller/1
  PID Controller/1 -> Out1/1
  vdc ref/1 -> Sum/2
  vdc/1 -> Sum/1

== system MicrogridControl/Solar/Solar Plant Integrated1/Detailed/PV Plant & Controller/Controller/Power Reference/Power Reference Controller/Power Reference Controller/Reference Current/Current limits ==
  Imax : Inport
  iqref : Inport  Port=2
  idref : Inport  Port=3
  Constant8 : Constant  Value=0
  Constant9 : Constant  Value=0
  Scope : Scope
      settings: ActiveDisplayYMinimum=-0.15  ActiveDisplayYMaximum=1.35  DataLoggingVariableName=ScopeData3
  Scope1 : Scope
      settings: ActiveDisplayYMinimum=-0.08298  ActiveDisplayYMaximum=0.74678  DataLoggingVariableName=ScopeData4
  Sqrt : Sqrt
  Sqrt1 : Sqrt
  Square{1..4} (4 alike) : Math  Operator=square
  Step2 : Step  Time=0.01  SampleTime=Ts
  Step3 : Step  Time=0.01  SampleTime=Ts
  Sum6 : Sum  Inputs=|+-
  Sum9 : Sum  Inputs=|+-
  Switch1 : Switch  Threshold=.01  SaturateOnIntegerOverflow=off  InputSameDT=off
  Switch2 : Switch  Threshold=.01  SaturateOnIntegerOverflow=off  InputSameDT=off
  iubq : Outport
  iubd : Outport  Port=2
  wires:
  idref/1 -> Square4/1
  Sqrt1/1 -> iubq/1, Scope1/1
  Imax/1 -> Square1/1, Square3/1
  Sqrt/1 -> iubd/1, Scope/1
  Constant9/1 -> Switch2/3
  Square4/1 -> Sum9/2
  Constant8/1 -> Switch1/3
  Square2/1 -> Sum6/2
  Sum6/1 -> Switch1/1
  Square3/1 -> Sum9/1
  iqref/1 -> Square2/1
  Switch1/1 -> Sqrt/1
  Square1/1 -> Sum6/1
  Switch2/1 -> Sqrt1/1
  Step2/1 -> Switch1/2
  Step3/1 -> Switch2/2
  Sum9/1 -> Switch2/1

== system MicrogridControl/Solar/Solar Plant Integrated1/Detailed/PV Plant & Controller/Controller/Power Reference/Power Reference Controller/Power Reference Controller/Reference Current/Refernce id generation ==
  V_mag : Inport
  ubid : Inport  Port=2
  PRef : Inport  Port=3
  Divide : Product  Inputs=/*
  Gain6 : Gain  Gain=-1
  P/Q Priority : Switch  Criteria=u2 ~= 0  SaturateOnIntegerOverflow=off  InputSameDT=off
  Priority Mode : Constant  Value=P-2
  Saturation Dynamic2 : simulink/Discontinuities/Saturation Dynamic  OutMin=[]  OutMax=[]  OutDataTypeStr=Inherit: Same as second input  OutDataType=fixdt(1, 16)  OutScaling=2^-10  DoSatur=off
  Saturation1 : Saturate  UpperLimit=Imax  LowerLimit=-Imax
  Scope : Scope
      settings: ActiveDisplayYMinimum=0.99583  ActiveDisplayYMaximum=1.02853
  Scope1 : Scope
      settings: ActiveDisplayYMinimum=-0.12499  ActiveDisplayYMaximum=1.12489  DataLoggingVariableName=ScopeData2
  ubid1 : InportShadow  Port=2
  id_ref : Outport
  wires:
  Divide/1 -> Saturation1/1, Saturation Dynamic2/2
  V_mag/1 -> Divide/1
  P/Q Priority/1 -> id_ref/1, Scope/1
  ubid1/1 -> Gain6/1
  Saturation1/1 -> P/Q Priority/1
  Priority Mode/1 -> P/Q Priority/2
  Saturation Dynamic2/1 -> P/Q Priority/3, Scope1/1
  Gain6/1 -> Saturation Dynamic2/3
  ubid/1 -> Saturation Dynamic2/1
  PRef/1 -> Divide/2

== system MicrogridControl/Solar/Solar Plant Integrated1/Detailed/PV Plant & Controller/Controller/Power Reference/Power Reference Controller/Power Reference Controller/Reference Current/Refernce iq generation ==
  ubiq : Inport
  V_mag : Inport  Port=2
  LVRT_iq : Inport  Port=3
  Q_ref : Inport  Port=4
  Divide1 : Product  Inputs=*/
  Gain : Gain  Gain=-1
  Gain1 : Gain  Gain=-1
  Gain7 : Gain  Gain=-1
  LVRT Priority : Switch  Threshold=.9  SaturateOnIntegerOverflow=off  InputSameDT=off
  P/Q Priority : Switch  Criteria=u2 ~= 0  SaturateOnIntegerOverflow=off  InputSameDT=off
  Priority Mode : Constant  Value=P-2
  Saturation Dynamic : simulink/Discontinuities/Saturation Dynamic  OutMin=[]  OutMax=[]  OutDataTypeStr=Inherit: Same as second input  OutDataType=fixdt(1, 16)  OutScaling=2^-10  DoSatur=off
  Saturation2 : Saturate  UpperLimit=1  LowerLimit=-1
  Saturation3 : Saturate  UpperLimit=Imax  LowerLimit=-Imax
  Scope : Scope  NumInputPorts=3
      settings: ActiveDisplayYMinimum=-0.025  ActiveDisplayYMaximum=0.22499  DataLoggingVariableName=ScopeData10
  ubiq1 : InportShadow
  iq_ref : Outport
  wires:
  Gain/1 -> iq_ref/1
  V_mag/1 -> Divide1/2, LVRT Priority/2
  Q_ref/1 -> Divide1/1
  ubiq1/1 -> Gain7/1
  LVRT_iq/1 -> Saturation2/1
  Gain7/1 -> Saturation Dynamic/3
  Saturation Dynamic/1 -> P/Q Priority/1
  Divide1/1 -> Saturation Dynamic/2, Saturation3/1
  Priority Mode/1 -> P/Q Priority/2
  Saturation3/1 -> P/Q Priority/3
  Saturation2/1 -> Gain1/1
  ubiq/1 -> Saturation Dynamic/1
  Gain1/1 -> LVRT Priority/3
  P/Q Priority/1 -> Scope/1, LVRT Priority/1
  LVRT Priority/1 -> Gain/1

== system MicrogridControl/Wind Farm/Wind Plant Integrated/Detailed/Wind Turbine and Converters/Wind Controller/Wind Grid-side Converter Controller/DC voltage controller & current reference/Subsystem1/V_dc_Controller1/PI ==
  Input : Inport
  Discrete-Time Integrator : DiscreteIntegrator  gainval=Ki_dc  SampleTime=Ts  ICPrevOutput=DiscIntNeverNeededParam  ICPrevScaledInput=DiscIntNeverNeededParam
  Gain1 : Gain  Gain=Kp_dc
  Sum1 : Sum  Inputs=|++
  Unit Delay : UnitDelay  SampleTime=Ts  HasFrameUpgradeWarning=on
  Out2 : Outport
  wires:
  Input/1 -> Discrete-Time Integrator/1, Gain1/1
  Gain1/1 -> Unit Delay/1
  Unit Delay/1 -> Sum1/2
  Sum1/1 -> Out2/1
  Discrete-Time Integrator/1 -> Sum1/1
